simulink model "Challenge1_1_1639535783"  (R2021a)
settings: Solver=VariableStepAuto  StartTime=0.0  StopTime=10.0  RelTol=1e-3
libraries: simulink x1
settings Model: Creator=Ish  LastModifiedBy=Ish

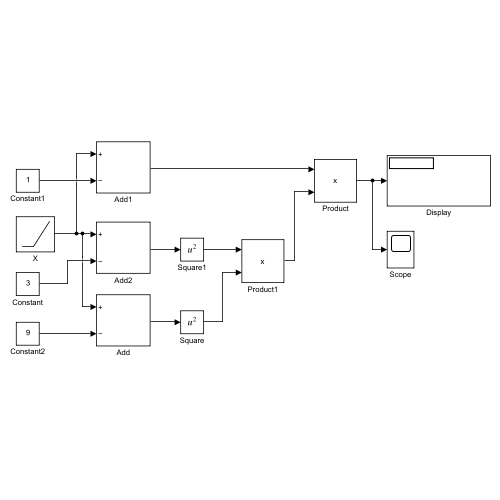
[thumbnail: Simulink's stored preview of the top-level diagram]
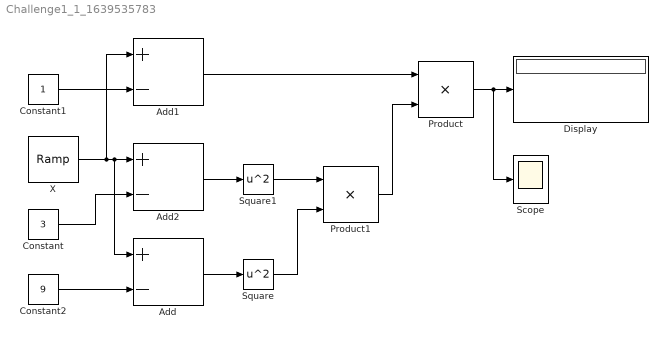
== system Challenge1_1_1639535783 ==
  Add : Sum  Inputs=+-
  Add1 : Sum  Inputs=+-
  Add2 : Sum  Inputs=+-
  Constant : Constant  Value=3
  Constant1 : Constant
  Constant2 : Constant  Value=9
  Display : Display
  Product : Product
  Product1 : Product
  Scope : Scope
  Square : Math  Operator=square  SaturateOnIntegerOverflow=on
  Square1 : Math  Operator=square  SaturateOnIntegerOverflow=on
  X : simulink/Sources/Ramp  slope=1  start=0  InitialOutput=0
  wires:
  Constant/1 -> Add2/2
  Add1/1 -> Product/1
  Square1/1 -> Product1/1
  Product/1 -> Scope/1, Display/1
  Square/1 -> Product1/2
  Constant1/1 -> Add1/2
  Product1/1 -> Product/2
  Constant2/1 -> Add/2
  Add2/1 -> Square1/1
  Add/1 -> Square/1
  X/1 -> Add2/1, Add/1, Add1/1
